simulink model "model"  (R2026a)
settings: Solver=VariableStepAuto  StopTime=6000  MaxStep=0.01  RelTol=1e-5
InitFcn:
  | init
values from neighbouring files (symbols this model uses):
  Bo = mo / (Ro*1000)^3    (= 2.23917907759e-05)    [init.m]
  d = [0 0 0.005]'    [init.m]
  inc = 30*pi/180    (= 0.523598775598)    [init.m]
  Ix = 0.029    [init.m]
  Iy = 0.024    [init.m]
  Iz = 0.005    [init.m]
  K_phi = 4.1144e-6    (= 4.1144e-06)    [init.m]
  K_psi = 2.5564e-6    (= 2.5564e-06)    [init.m]
  K_theta = 3.0000e-6    (= 3e-06)    [init.m]
  mu = 3.986e5    (= 398600)    [init.m]
  q_ic = [0 0 0 1]'    [init.m]
  Ro = Re+h    (= 7078)    [init.m]
  T1_phi = 300    [init.m]
  T1_psi = 300    [init.m]
  T1_theta = 300    [init.m]
  T2_phi = 12    [init.m]
  T2_psi = 7    [init.m]
  T2_theta = 7    [init.m]
  w0 = sqrt(mu/(Ro^3))    [init.m]
  w_bi_ic = w_oi    [init.m]
  w_oi = [0 -w0 0]'    [init.m]
libraries: matrix_library x1
settings Model: Creator=demleo23082  LastModifiedBy=User

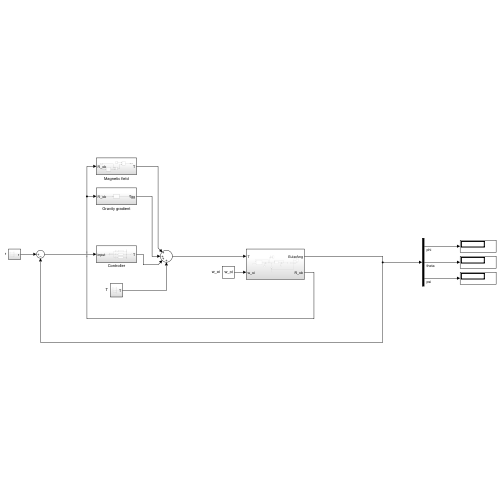
[thumbnail: Simulink's stored preview of the top-level diagram]
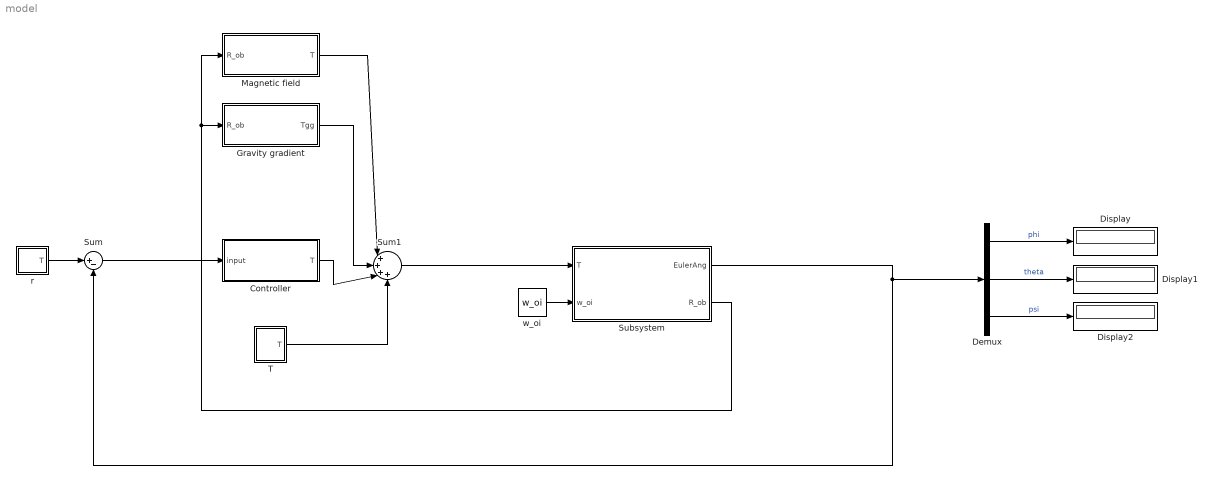
== system model ==
  Controller : Subsystem
  Demux : Demux  Outputs=3
  Display : Display
  Display1 : Display
  Display2 : Display
  Gravity gradient : Subsystem
  Magnetic field : Subsystem
  Subsystem : Subsystem
  Sum : Sum  Inputs=|+-
  Sum1 : Sum  Inputs=|++++
  T : Subsystem
  r : Subsystem
  w_oi : Constant  Value=w_oi  VectorParams1D=off
  wires:
  w_oi/1 -> Subsystem/2(w_oi)
  r/1(T) -> Sum/1
  Sum/1 -> Controller/1(input)
  Subsystem/1(EulerAng) -> Demux/1, Sum/2
  Sum1/1 -> Subsystem/1(T)
  Controller/1(T) -> Sum1/3
  Demux/1 -> Display/1  "phi"
  Demux/2 -> Display1/1  "theta"
  Demux/3 -> Display2/1  "psi"
  T/1(T) -> Sum1/4
  Subsystem/2(R_ob) -> Gravity gradient/1(R_ob), Magnetic field/1(R_ob)
  Gravity gradient/1(Tgg) -> Sum1/2
  Magnetic field/1(T) -> Sum1/1

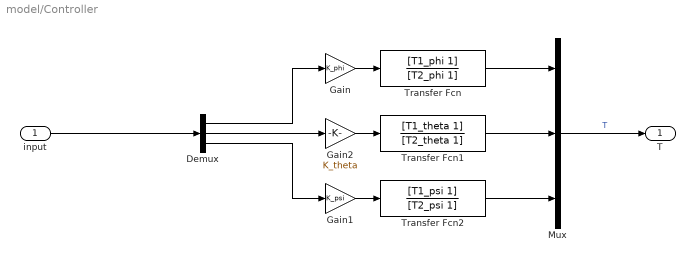
== system model/Controller ==
  input : Inport
  Demux : Demux  Outputs=3
  Gain : Gain  Gain=K_phi
  Gain1 : Gain  Gain=K_psi
  Gain2 : Gain  Gain=K_theta
  Mux : Mux  Inputs=3
  Transfer Fcn : TransferFcn  Numerator=[T1_phi 1]  Denominator=[T2_phi 1]
  Transfer Fcn1 : TransferFcn  Numerator=[T1_theta 1]  Denominator=[T2_theta 1]
  Transfer Fcn2 : TransferFcn  Numerator=[T1_psi 1]  Denominator=[T2_psi 1]
  T : Outport
  wires:
  Demux/3 -> Gain1/1
  Transfer Fcn/1 -> Mux/1
  Transfer Fcn1/1 -> Mux/2
  Demux/2 -> Gain2/1
  Mux/1 -> T/1  "T"
  input/1 -> Demux/1
  Transfer Fcn2/1 -> Mux/3
  Demux/1 -> Gain/1
  Gain/1 -> Transfer Fcn/1
  Gain2/1 -> Transfer Fcn1/1
  Gain1/1 -> Transfer Fcn2/1

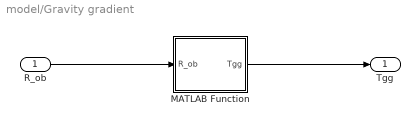
== system model/Gravity gradient ==
  R_ob : Inport
  MATLAB Function : MATLAB Function  TreatAsAtomicUnit=on
  Tgg : Outport
  wires:
  R_ob/1 -> MATLAB Function/1(R_ob)
  MATLAB Function/1(Tgg) -> Tgg/1

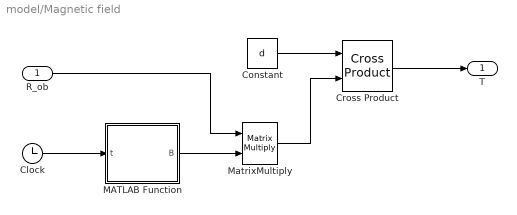
== system model/Magnetic field ==
  R_ob : Inport
  Clock : Clock
  Constant : Constant  Value=d
  Cross Product : matrix_library/Cross Product
  MATLAB Function : MATLAB Function  TreatAsAtomicUnit=on
  MatrixMultiply : Product  Multiplication=Matrix(*)
  T : Outport
  wires:
  R_ob/1 -> MatrixMultiply/1
  Clock/1 -> MATLAB Function/1(t)
  MATLAB Function/1(B) -> MatrixMultiply/2
  Constant/1 -> Cross Product/1
  MatrixMultiply/1 -> Cross Product/2
  Cross Product/1 -> T/1

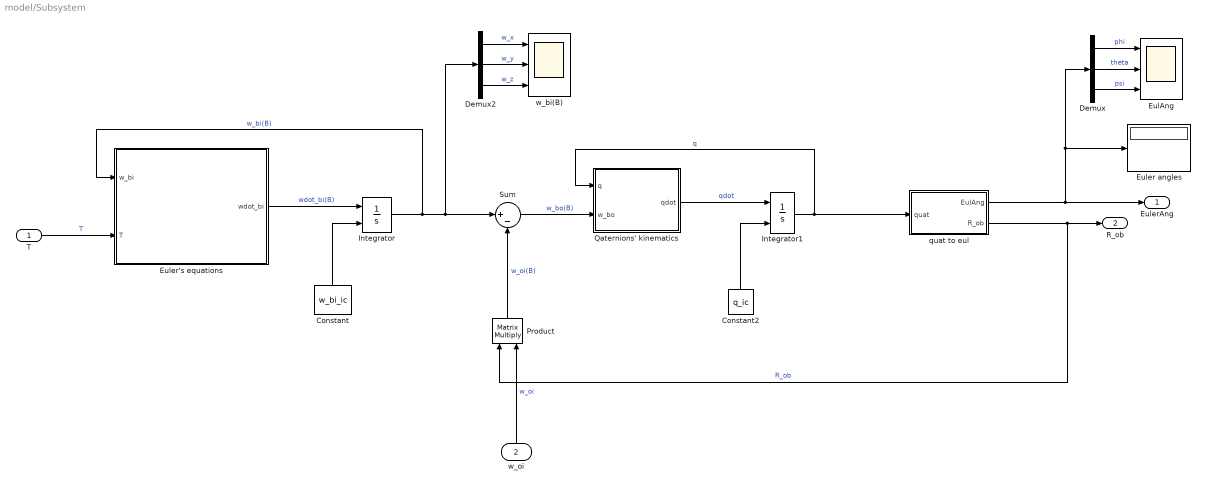
== system model/Subsystem ==
  T : Inport
  w_oi : Inport  Port=2
  Constant : Constant  Value=w_bi_ic  VectorParams1D=off
  Constant2 : Constant  Value=q_ic  VectorParams1D=off
  Demux : Demux  Outputs=3
  Demux2 : Demux  Outputs=3
  EulAng : Scope  NumInputPorts=3
      settings: ActiveDisplayString=3  ActiveDisplayYMinimum=-0.58513829595827138  ActiveDisplayYMaximum=0.37409833435583789
  Euler angles : Display
  Euler's equations : MATLAB Function  TreatAsAtomicUnit=on
  Integrator : Integrator  InitialConditionSource=external
  Integrator1 : Integrator  InitialConditionSource=external
  Product : Product  Multiplication=Matrix(*)
  Qaternions' kinematics : MATLAB Function  TreatAsAtomicUnit=on
  Sum : Sum  Inputs=|+-
  quat to eul : Subsystem
  w_bi(B) : Scope  NumInputPorts=3
      settings: ActiveDisplayYMinimum=-0.0085250800491360919  ActiveDisplayYMaximum=0.002573853184285815
  EulerAng : Outport
  R_ob : Outport  Port=2
  wires:
  Integrator/1 -> Sum/1, Demux2/1, Euler's equations/1(w_bi)  "w_bi(B)"
  Constant2/1 -> Integrator1/2
  Integrator1/1 -> quat to eul/1(quat), Qaternions' kinematics/1(q)  "q"
  Product/1 -> Sum/2  "w_oi(B)"
  quat to eul/2(R_ob) -> Product/1, R_ob/1  "R_ob"
  Sum/1 -> Qaternions' kinematics/2(w_bo)  "w_bo(B)"
  Euler's equations/1(wdot_bi) -> Integrator/1  "wdot_bi(B)"
  Qaternions' kinematics/1(qdot) -> Integrator1/1  "qdot"
  quat to eul/1(EulAng) -> Euler angles/1, Demux/1, EulerAng/1
  Demux/1 -> EulAng/1  "phi"
  Demux/3 -> EulAng/3  "psi"
  Demux/2 -> EulAng/2  "theta"
  w_oi/1 -> Product/2  "w_oi"
  Constant/1 -> Integrator/2
  T/1 -> Euler's equations/2(T)  "T"
  Demux2/1 -> w_bi(B)/1  "w_x"
  Demux2/2 -> w_bi(B)/2  "w_y"
  Demux2/3 -> w_bi(B)/3  "w_z"

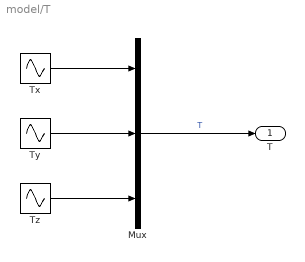
== system model/T ==
  Mux : Mux  Inputs=3
  Tx : Sin  Amplitude=8e-08  Frequency=1e-3  Phase=pi/2  SampleTime=0
  Ty : Sin  Amplitude=4e-08  Frequency=1e-3  Phase=pi/2  SampleTime=0
  Tz : Sin  Amplitude=2e-08  Frequency=1e-3  Phase=pi/2  SampleTime=0
  T : Outport
  wires:
  Tx/1 -> Mux/1
  Tz/1 -> Mux/3
  Ty/1 -> Mux/2
  Mux/1 -> T/1  "T"

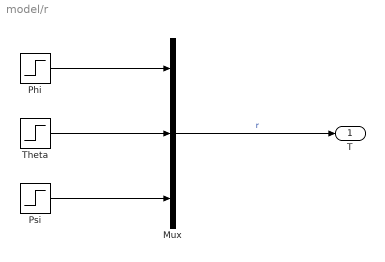
== system model/r ==
  Mux : Mux  Inputs=3
  Phi : Step  Time=200  FinalValue=20*pi/180  SampleTime=0
  Psi : Step  Time=0  FinalValue=0  SampleTime=0
  Theta : Step  Time=0  FinalValue=0  SampleTime=0
  T : Outport
  wires:
  Mux/1 -> T/1  "r"
  Theta/1 -> Mux/2
  Psi/1 -> Mux/3
  Phi/1 -> Mux/1

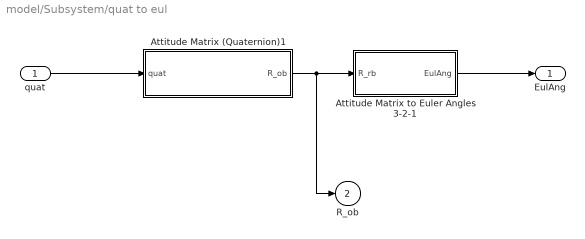
== system model/Subsystem/quat to eul ==
  quat : Inport
  Attitude Matrix (Quaternion)1 : Subsystem
  Attitude Matrix to Euler Angles 3-2-1 : Subsystem
  EulAng : Outport  VectorParamsAs1DForOutWhenUnconnected=off
  R_ob : Outport  Port=2
  wires:
  Attitude Matrix to Euler Angles 3-2-1/1(EulAng) -> EulAng/1
  Attitude Matrix (Quaternion)1/1(R_ob) -> Attitude Matrix to Euler Angles 3-2-1/1(R_rb), R_ob/1
  quat/1 -> Attitude Matrix (Quaternion)1/1(quat)

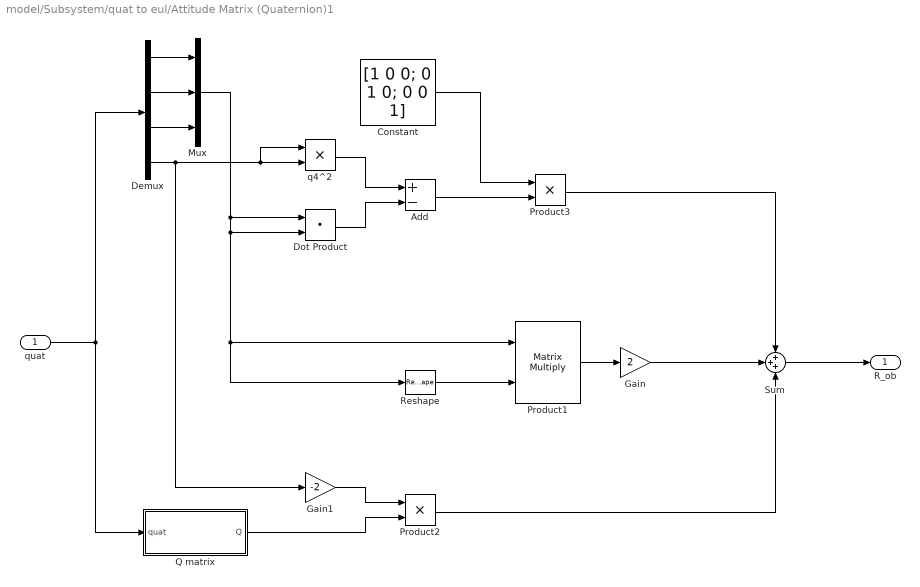
== system model/Subsystem/quat to eul/Attitude Matrix (Quaternion)1 ==
  quat : Inport
  Add : Sum  Inputs=+-
  Constant : Constant  Value=[1 0 0; 0 1 0; 0 0 1]
  Demux : Demux
  Dot Product : DotProduct  OutDataTypeStr=Inherit: Inherit via internal rule
  Gain : Gain  Gain=2
  Gain1 : Gain  Gain=-2
  Mux : Mux  Inputs=3
  Product1 : Product  Multiplication=Matrix(*)  RndMeth=Zero
  Product2 : Product  RndMeth=Zero
  Product3 : Product  RndMeth=Zero
  Q matrix : Subsystem
  Reshape : Reshape  OutputDimensionality=Row vector (2-D)
  Sum : Sum  Inputs=+++
  q4^2 : Product  RndMeth=Zero
  R_ob : Outport  VectorParamsAs1DForOutWhenUnconnected=off
  wires:
  quat/1 -> Demux/1, Q matrix/1(quat)
  Demux/4 -> q4^2/2, q4^2/1, Gain1/1
  Reshape/1 -> Product1/2
  Product1/1 -> Gain/1
  Gain/1 -> Sum/2
  q4^2/1 -> Add/1
  Dot Product/1 -> Add/2
  Product2/1 -> Sum/3
  Add/1 -> Product3/2
  Sum/1 -> R_ob/1
  Constant/1 -> Product3/1
  Product3/1 -> Sum/1
  Demux/1 -> Mux/1
  Demux/2 -> Mux/2
  Demux/3 -> Mux/3
  Mux/1 -> Dot Product/1, Reshape/1, Product1/1, Dot Product/2
  Gain1/1 -> Product2/1
  Q matrix/1(Q) -> Product2/2

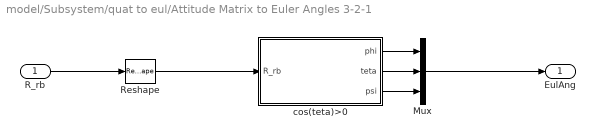
== system model/Subsystem/quat to eul/Attitude Matrix to Euler Angles 3-2-1 ==
  R_rb : Inport
  Mux : Mux  Inputs=3
  Reshape : Reshape  OutputDimensionality=Column vector (2-D)
  cos(teta)>0 : Subsystem
  EulAng : Outport  VectorParamsAs1DForOutWhenUnconnected=off
  wires:
  cos(teta)>0/2(teta) -> Mux/2
  cos(teta)>0/1(phi) -> Mux/1
  cos(teta)>0/3(psi) -> Mux/3
  Mux/1 -> EulAng/1
  Reshape/1 -> cos(teta)>0/1(R_rb)
  R_rb/1 -> Reshape/1

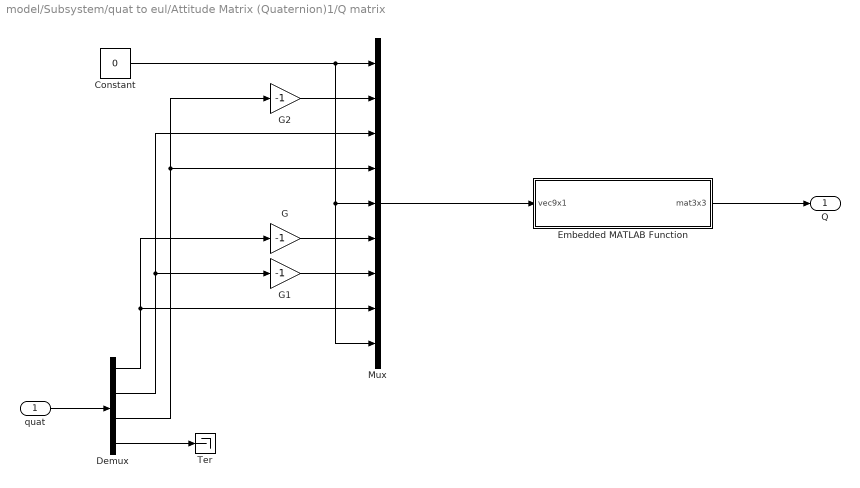
== system model/Subsystem/quat to eul/Attitude Matrix (Quaternion)1/Q matrix ==
  quat : Inport
  Constant : Constant  Value=0
  Demux : Demux
  Embedded MATLAB Function : MATLAB Function  TreatAsAtomicUnit=on
  G : Gain  Gain=-1
  G1 : Gain  Gain=-1
  G2 : Gain  Gain=-1
  Mux : Mux  Inputs=9
  Ter : Terminator
  Q : Outport  VectorParamsAs1DForOutWhenUnconnected=off
  wires:
  Demux/4 -> Ter/1
  quat/1 -> Demux/1
  Constant/1 -> Mux/9, Mux/5, Mux/1
  Demux/1 -> G/1, Mux/8
  G1/1 -> Mux/7
  Demux/2 -> G1/1, Mux/3
  G/1 -> Mux/6
  G2/1 -> Mux/2
  Demux/3 -> G2/1, Mux/4
  Embedded MATLAB Function/1(mat3x3) -> Q/1
  Mux/1 -> Embedded MATLAB Function/1(vec9x1)

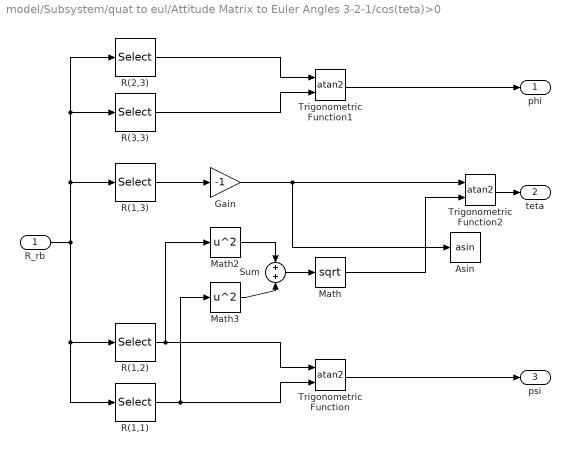
== system model/Subsystem/quat to eul/Attitude Matrix to Euler Angles 3-2-1/cos(teta)>0 ==
  R_rb : Inport
  Asin : Trigonometry  Operator=asin
  Gain : Gain  Gain=-1
  Math : Math  Operator=sqrt  SignedPower=on
  Math2 : Math  Operator=square  SignedPower=on
  Math3 : Math  Operator=square  SignedPower=on
  R(1,1) : Selector  InputPortWidth=9  IndexOptions=Index vector (dialog)  Indices=[1]  OutputSizes=1
  R(1,2) : Selector  InputPortWidth=9  IndexOptions=Index vector (dialog)  Indices=[4]  OutputSizes=1
  R(1,3) : Selector  InputPortWidth=9  IndexOptions=Index vector (dialog)  Indices=[7]  OutputSizes=1
  R(2,3) : Selector  InputPortWidth=9  IndexOptions=Index vector (dialog)  Indices=[8]  OutputSizes=1
  R(3,3) : Selector  InputPortWidth=9  IndexOptions=Index vector (dialog)  Indices=[9]  OutputSizes=1
  Sum : Sum
  Trigonometric Function : Trigonometry  Operator=atan2
  Trigonometric Function1 : Trigonometry  Operator=atan2
  Trigonometric Function2 : Trigonometry  Operator=atan2
  phi : Outport  VectorParamsAs1DForOutWhenUnconnected=off
  teta : Outport  Port=2  VectorParamsAs1DForOutWhenUnconnected=off
  psi : Outport  Port=3  VectorParamsAs1DForOutWhenUnconnected=off
  wires:
  R_rb/1 -> R(1,1)/1, R(1,2)/1, R(1,3)/1, R(3,3)/1, R(2,3)/1
  R(1,2)/1 -> Trigonometric Function/1, Math2/1
  R(1,1)/1 -> Trigonometric Function/2, Math3/1
  R(2,3)/1 -> Trigonometric Function1/1
  R(3,3)/1 -> Trigonometric Function1/2
  R(1,3)/1 -> Gain/1
  Gain/1 -> Asin/1, Trigonometric Function2/1
  Math2/1 -> Sum/1
  Math3/1 -> Sum/2
  Sum/1 -> Math/1
  Math/1 -> Trigonometric Function2/2
  Trigonometric Function1/1 -> phi/1
  Trigonometric Function2/1 -> teta/1
  Trigonometric Function/1 -> psi/1

== matlab function model/Subsystem/Qaternions' kinematics ==
  data: q input; w_bo input; qdot output
function qdot = fcn(q, w_bo)

%--------------------------------------------------------------------------

% Computes quaternion derivative from body angular velocity

%--------------------------------------------------------------------------

% Extract angular velocity components

Wx = w_bo(1);
Wy = w_bo(2);
Wz = w_bo(3);

%--------------------------------------------------------------------------

% Quaternion kinematic matrix

Q = [0 Wz -Wy Wx; -Wz 0 Wx Wy; Wy -Wx 0 Wz; -Wx -Wy -Wz 0];

%--------------------------------------------------------------------------

% Quaternion derivative

qdot = 0.5 * Q * q;

%--------------------------------------------------------------------------

== matlab function model/Subsystem/Euler's equations ==
  data: w_bi input; T input; wdot_bi output; Ix parameter; Iy parameter; Iz parameter
function wdot_bi = fcn(w_bi, T, Ix, Iy, Iz)

%--------------------------------------------------------------------------

% Computes angular acceleration of the body (b) wrt inertial frame (i)
% using Euler’s rotational dynamics equations

%--------------------------------------------------------------------------

% Individual components of angular acceleration

wdot_bi_x = - w_bi(2) * w_bi(3) * (Iz - Iy) / Ix + T(1) / Ix;

wdot_bi_y = - w_bi(1) * w_bi(3) * (Ix - Iz) / Iy + T(2) / Iy;

wdot_bi_z = - w_bi(1) * w_bi(2) * (Iy - Ix) / Iz + T(3) / Iz;

%--------------------------------------------------------------------------

% Output angular acceleration vector

wdot_bi = [wdot_bi_x wdot_bi_y wdot_bi_z]';

%--------------------------------------------------------------------------

== matlab function model/Subsystem/quat to eul/Attitude Matrix (Quaternion)1/Q matrix/Embedded MATLAB Function ==
  data: vec9x1 input; mat3x3 output
function mat3x3 = vec2mat(vec9x1)
%#eml

s = size(vec9x1);

if s(1)>s(2)
    vec = vec9x1';
else
    vec = vec9x1;
end

mat3x3 = [vec(1:3); vec(4:6); vec(7:9)];

== matlab function model/Gravity gradient/MATLAB Function ==
  data: R_ob input; Tgg output; mu parameter; Ro parameter; Ix parameter; Iy parameter; Iz parameter
function Tgg = fcn(R_ob, mu, Ro, Ix, Iy, Iz)

Tgg_x = ((3*mu)/Ro^3)*abs(Iz-Iy)*R_ob(2,3)*R_ob(3,3);
Tgg_y = -((3*mu)/Ro^3)*abs(Iz-Ix)*R_ob(1,3)*R_ob(3,3);
Tgg_z = -((3*mu)/Ro^3)*abs(Ix-Iy)*R_ob(1,3)*R_ob(2,3);

Tgg = [Tgg_x Tgg_y Tgg_z]';

== matlab function model/Magnetic field/MATLAB Function ==
  data: B output; t input; Bo parameter; inc parameter; w0 parameter
function B = fcn(t, Bo, inc, w0)

Bo_x = Bo * cos(inc * sin(w0 * t)) * sin(inc * cos(w0 * t));
Bo_y = -Bo * cos(inc * sin(w0 * t)) * cos(inc * cos(w0 * t));
Bo_z = 2* Bo * sin(inc * cos(w0 * t));

B = [Bo_x Bo_y Bo_z]';
